simulink model "planta_controlador_integrados_rev_0"  (R2022a)
settings: Solver=ode1  StartTime=0.0  StopTime=tfinal  FixedStep=tstep  RelTol=1e-3
undefined symbols (not defined in the file or in its folder): wp_index_lim, wp_lat, wp_long, wp_time
settings Model: Creator=rodri  LastModifiedBy=rodri
settings DataIOCC: ExternalInput=[t2, u2]  SaveFormat=StructureWithTime  SignalLogging=off  DSMLogging=off  InspectSignalLogs=on  ReturnWorkspaceOutputs=off

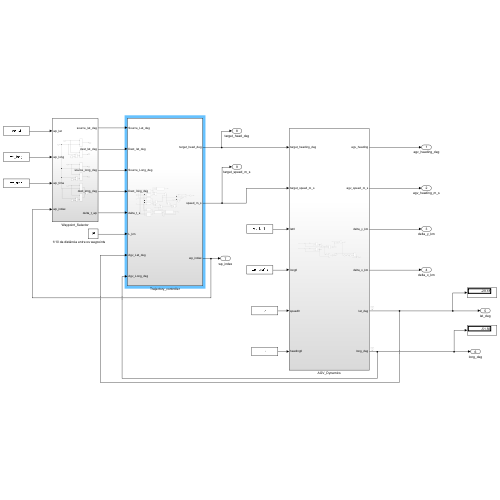
[thumbnail: Simulink's stored preview of the top-level diagram]
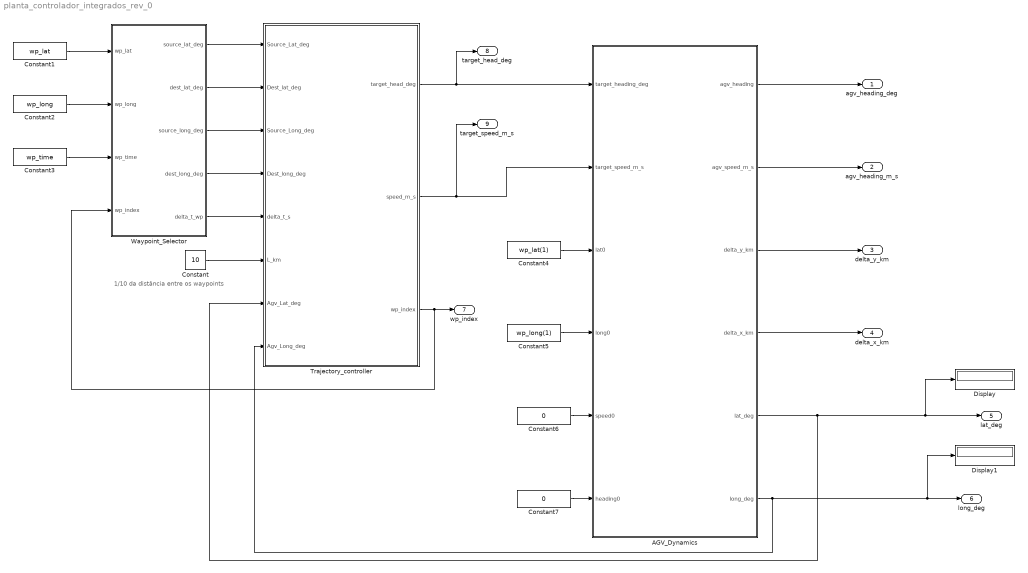
== system planta_controlador_integrados_rev_0 ==
  note: 1/10 da distância entre os waypoints
  AGV_Dynamics : Subsystem
  Constant : Constant  Value=10
  Constant1 : Constant  Value=wp_lat
  Constant2 : Constant  Value=wp_long
  Constant3 : Constant  Value=wp_time
  Constant4 : Constant  Value=wp_lat(1)
  Constant5 : Constant  Value=wp_long(1)
  Constant6 : Constant  Value=0
  Constant7 : Constant  Value=0
  Display : Display
  Display1 : Display
  Trajectory_controller : Subsystem
  Waypoint_Selector : Subsystem
  agv_heading_deg : Outport
  agv_heading_m_s : Outport  Port=2
  delta_y_km : Outport  Port=3
  delta_x_km : Outport  Port=4
  lat_deg : Outport  Port=5
  long_deg : Outport  Port=6
  wp_index : Outport  Port=7
  target_head_deg : Outport  Port=8
  target_speed_m_s : Outport  Port=9
  wires:
  Waypoint_Selector/1(source_lat_deg) -> Trajectory_controller/1(Source_Lat_deg)
  Waypoint_Selector/2(dest_lat_deg) -> Trajectory_controller/2(Dest_lat_deg)
  Waypoint_Selector/3(source_long_deg) -> Trajectory_controller/3(Source_Long_deg)
  Waypoint_Selector/4(dest_long_deg) -> Trajectory_controller/4(Dest_long_deg)
  Constant/1 -> Trajectory_controller/6(L_km)
  Constant1/1 -> Waypoint_Selector/1(wp_lat)
  Constant2/1 -> Waypoint_Selector/2(wp_long)
  Constant3/1 -> Waypoint_Selector/3(wp_time)
  Waypoint_Selector/5(delta_t_wp) -> Trajectory_controller/5(delta_t_s)
  Trajectory_controller/3(wp_index) -> Waypoint_Selector/4(wp_index), wp_index/1
  Trajectory_controller/1(target_head_deg) -> target_head_deg/1, AGV_Dynamics/1(target_heading_deg)
  Trajectory_controller/2(speed_m_s) -> AGV_Dynamics/2(target_speed_m_s), target_speed_m_s/1
  AGV_Dynamics/5(lat_deg) -> Display/1, lat_deg/1, Trajectory_controller/7(Agv_Lat_deg)
  AGV_Dynamics/6(long_deg) -> Display1/1, long_deg/1, Trajectory_controller/8(Agv_Long_deg)
  AGV_Dynamics/1(agv_heading) -> agv_heading_deg/1
  AGV_Dynamics/2(agv_speed_m_s) -> agv_heading_m_s/1
  AGV_Dynamics/3(delta_y_km) -> delta_y_km/1
  AGV_Dynamics/4(delta_x_km) -> delta_x_km/1
  Constant4/1 -> AGV_Dynamics/3(lat0)
  Constant5/1 -> AGV_Dynamics/4(long0)
  Constant6/1 -> AGV_Dynamics/5(speed0)
  Constant7/1 -> AGV_Dynamics/6(heading0)

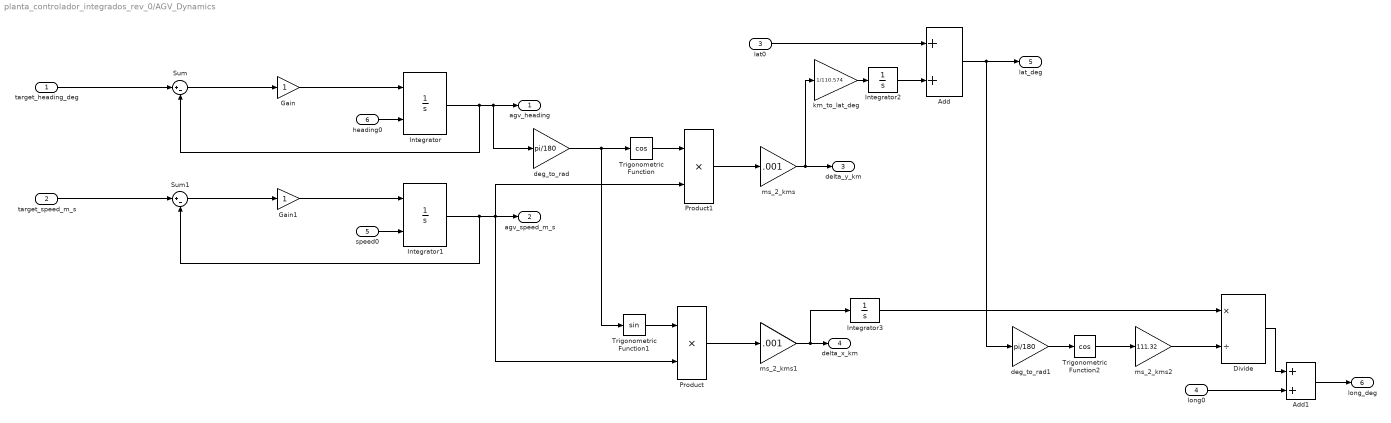
== system planta_controlador_integrados_rev_0/AGV_Dynamics ==
  target_heading_deg : Inport
  target_speed_m_s : Inport  Port=2
  lat0 : Inport  Port=3
  long0 : Inport  Port=4
  speed0 : Inport  Port=5
  heading0 : Inport  Port=6
  Add : Sum
  Add1 : Sum
  Divide : Product  Inputs=*/
  Gain : Gain
  Gain1 : Gain
  Integrator : Integrator  InitialConditionSource=external
  Integrator1 : Integrator  InitialConditionSource=external
  Integrator2 : Integrator
  Integrator3 : Integrator
  Product : Product
  Product1 : Product
  Sum : Sum  Inputs=|+-
  Sum1 : Sum  Inputs=|+-
  Trigonometric Function : Trigonometry  Operator=cos
  Trigonometric Function1 : Trigonometry
  Trigonometric Function2 : Trigonometry  Operator=cos
  deg_to_rad : Gain  Gain=pi/180
  deg_to_rad1 : Gain  Gain=pi/180
  km_to_lat_deg : Gain  Gain=1/110.574
  ms_2_kms : Gain  Gain=.001
  ms_2_kms1 : Gain  Gain=.001
  ms_2_kms2 : Gain  Gain=111.32
  agv_heading : Outport
  agv_speed_m_s : Outport  Port=2
  delta_y_km : Outport  Port=3
  delta_x_km : Outport  Port=4
  lat_deg : Outport  Port=5
  long_deg : Outport  Port=6
  wires:
  Integrator/1 -> Sum/2, deg_to_rad/1, agv_heading/1
  Gain/1 -> Integrator/1
  Sum/1 -> Gain/1
  target_heading_deg/1 -> Sum/1
  target_speed_m_s/1 -> Sum1/1
  Gain1/1 -> Integrator1/1
  Sum1/1 -> Gain1/1
  Integrator1/1 -> Sum1/2, Product1/2, Product/2, agv_speed_m_s/1
  heading0/1 -> Integrator/2
  speed0/1 -> Integrator1/2
  deg_to_rad/1 -> Trigonometric Function1/1, Trigonometric Function/1
  Trigonometric Function1/1 -> Product/1
  Product/1 -> ms_2_kms1/1
  Trigonometric Function/1 -> Product1/1
  Product1/1 -> ms_2_kms/1
  ms_2_kms/1 -> delta_y_km/1, km_to_lat_deg/1
  ms_2_kms1/1 -> Integrator3/1, delta_x_km/1
  lat0/1 -> Add/1
  km_to_lat_deg/1 -> Integrator2/1
  Add/1 -> deg_to_rad1/1, lat_deg/1
  deg_to_rad1/1 -> Trigonometric Function2/1
  Trigonometric Function2/1 -> ms_2_kms2/1
  long0/1 -> Add1/2
  Divide/1 -> Add1/1
  ms_2_kms2/1 -> Divide/2
  Add1/1 -> long_deg/1
  Integrator3/1 -> Divide/1
  Integrator2/1 -> Add/2

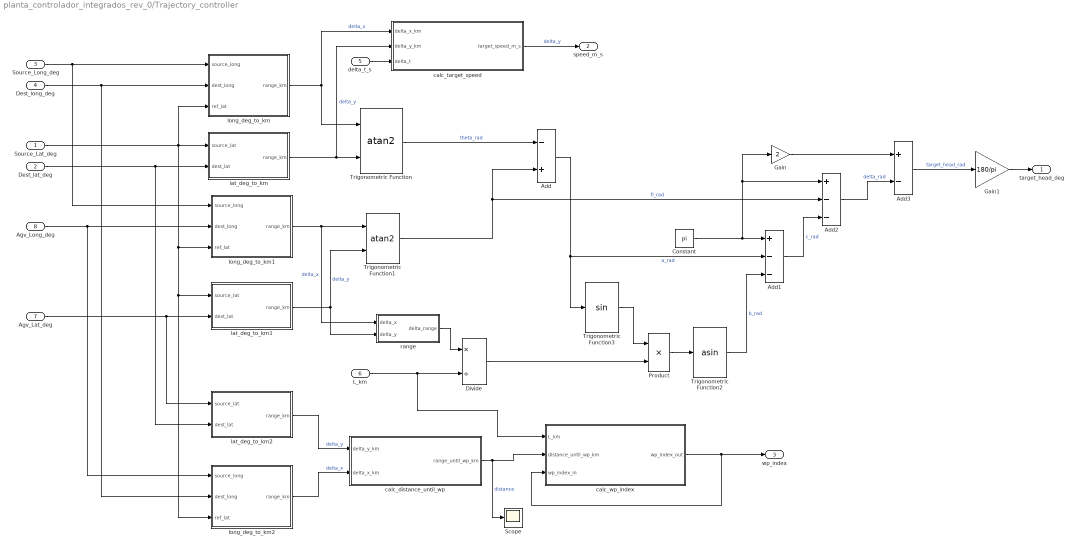
== system planta_controlador_integrados_rev_0/Trajectory_controller ==
  Source_Lat_deg : Inport
  Dest_lat_deg : Inport  Port=2
  Source_Long_deg : Inport  Port=3
  Dest_long_deg : Inport  Port=4
  delta_t_s : Inport  Port=5
  L_km : Inport  Port=6
  Agv_Lat_deg : Inport  Port=7
  Agv_Long_deg : Inport  Port=8
  Add : Sum  Inputs=-+
  Add1 : Sum  Inputs=+--
  Add2 : Sum  Inputs=+--
  Add3 : Sum  Inputs=+-
  Constant : Constant  Value=pi
  Divide : Product  Inputs=*/
  Gain : Gain  Gain=2
  Gain1 : Gain  Gain=180/pi
  Product : Product
  Scope : Scope
  Trigonometric Function : Trigonometry  Operator=atan2
  Trigonometric Function1 : Trigonometry  Operator=atan2
  Trigonometric Function2 : Trigonometry  Operator=asin
  Trigonometric Function3 : Trigonometry
  calc_distance_until_wp : Subsystem
  calc_target_speed : Subsystem
  calc_wp_index : Subsystem
  lat_deg_to_km : Subsystem
  lat_deg_to_km1 : Subsystem
  lat_deg_to_km2 : Subsystem
  long_deg_to_km : Subsystem
  long_deg_to_km1 : Subsystem
  long_deg_to_km2 : Subsystem
  range : Subsystem
  target_head_deg : Outport
  speed_m_s : Outport  Port=2
  wp_index : Outport  Port=3
  wires:
  Dest_lat_deg/1 -> lat_deg_to_km2/2(dest_lat), lat_deg_to_km/2(dest_lat)
  Source_Lat_deg/1 -> long_deg_to_km/3(ref_lat), long_deg_to_km2/3(ref_lat), lat_deg_to_km1/1(source_lat), long_deg_to_km1/3(ref_lat), lat_deg_to_km/1(source_lat)
  Agv_Lat_deg/1 -> lat_deg_to_km2/1(source_lat), lat_deg_to_km1/2(dest_lat)
  Source_Long_deg/1 -> long_deg_to_km1/1(source_long), long_deg_to_km/1(source_long)
  Dest_long_deg/1 -> long_deg_to_km/2(dest_long), long_deg_to_km2/2(dest_long)
  long_deg_to_km/1(range_km) -> calc_target_speed/1(delta_x_km), Trigonometric Function/1  "delta_x"
  lat_deg_to_km/1(range_km) -> calc_target_speed/2(delta_y_km), Trigonometric Function/2  "delta_y"
  Agv_Long_deg/1 -> long_deg_to_km2/1(source_long), long_deg_to_km1/2(dest_long)
  long_deg_to_km1/1(range_km) -> range/1(delta_x), Trigonometric Function1/1  "delta_x"
  lat_deg_to_km1/1(range_km) -> Trigonometric Function1/2, range/2(delta_y)  "delta_y"
  Trigonometric Function1/1 -> Add2/2, Add/2  "fi_rad"
  Trigonometric Function/1 -> Add/1  "theta_rad"
  Add/1 -> Add1/2, Trigonometric Function3/1  "a_rad"
  range/1(delta_range) -> Divide/1
  L_km/1 -> calc_wp_index/1(L_km), Divide/2
  Product/1 -> Trigonometric Function2/1
  Trigonometric Function3/1 -> Product/1
  Divide/1 -> Product/2
  Trigonometric Function2/1 -> Add1/3  "b_rad"
  Constant/1 -> Gain/1, Add2/1, Add1/1
  Add1/1 -> Add2/3  "c_rad"
  Add2/1 -> Add3/2  "delta_rad"
  Gain/1 -> Add3/1
  Add3/1 -> Gain1/1  "target_head_rad"
  Gain1/1 -> target_head_deg/1
  delta_t_s/1 -> calc_target_speed/3(delta_t)
  calc_target_speed/1(target_speed_m_s) -> speed_m_s/1  "delta_y"
  lat_deg_to_km2/1(range_km) -> calc_distance_until_wp/1(delta_y_km)  "delta_y"
  long_deg_to_km2/1(range_km) -> calc_distance_until_wp/2(delta_x_km)  "delta_x"
  calc_distance_until_wp/1(range_until_wp_km) -> Scope/1, calc_wp_index/2(distance_until_wp_km)  "distance"
  calc_wp_index/1(wp_index_out) -> calc_wp_index/3(wp_index_in), wp_index/1

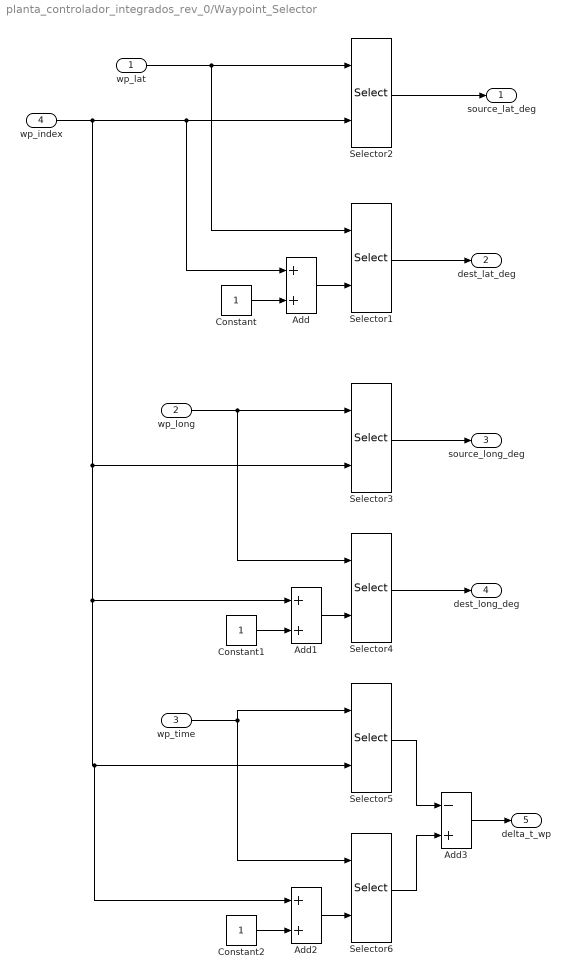
== system planta_controlador_integrados_rev_0/Waypoint_Selector ==
  wp_lat : Inport
  wp_long : Inport  Port=2
  wp_time : Inport  Port=3
  wp_index : Inport  Port=4
  Add : Sum
  Add1 : Sum
  Add2 : Sum
  Add3 : Sum  Inputs=-+
  Constant : Constant
  Constant1 : Constant
  Constant2 : Constant
  Selector{1..6} (6 alike) : Selector  InputPortWidth=num_of_wps  IndexOptions=Index vector (port)  Indices=[1 3]  OutputSizes=1
  source_lat_deg : Outport
  dest_lat_deg : Outport  Port=2
  source_long_deg : Outport  Port=3
  dest_long_deg : Outport  Port=4
  delta_t_wp : Outport  Port=5
  wires:
  Selector2/1 -> source_lat_deg/1
  Selector1/1 -> dest_lat_deg/1
  wp_lat/1 -> Selector2/1, Selector1/1
  Add/1 -> Selector1/2
  Constant/1 -> Add/2
  Selector3/1 -> source_long_deg/1
  Selector4/1 -> dest_long_deg/1
  wp_long/1 -> Selector4/1, Selector3/1
  Constant1/1 -> Add1/2
  Add1/1 -> Selector4/2
  Add2/1 -> Selector6/2
  Constant2/1 -> Add2/2
  wp_time/1 -> Selector5/1, Selector6/1
  wp_index/1 -> Add2/1, Selector5/2, Add1/1, Selector3/2, Selector2/2, Add/1
  Selector5/1 -> Add3/1
  Selector6/1 -> Add3/2
  Add3/1 -> delta_t_wp/1

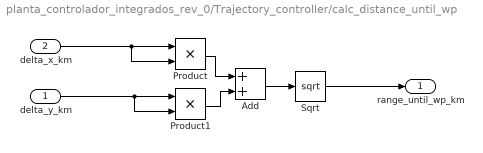
== system planta_controlador_integrados_rev_0/Trajectory_controller/calc_distance_until_wp ==
  delta_y_km : Inport
  delta_x_km : Inport  Port=2
  Add : Sum
  Product : Product
  Product1 : Product
  Sqrt : Sqrt
  range_until_wp_km : Outport
  wires:
  Sqrt/1 -> range_until_wp_km/1
  Product1/1 -> Add/2
  Product/1 -> Add/1
  Add/1 -> Sqrt/1
  delta_x_km/1 -> Product/1, Product/2
  delta_y_km/1 -> Product1/1, Product1/2

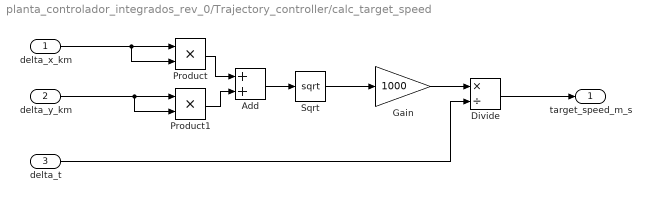
== system planta_controlador_integrados_rev_0/Trajectory_controller/calc_target_speed ==
  delta_x_km : Inport
  delta_y_km : Inport  Port=2
  delta_t : Inport  Port=3
  Add : Sum
  Divide : Product  Inputs=*/
  Gain : Gain  Gain=1000
  Product : Product
  Product1 : Product
  Sqrt : Sqrt
  target_speed_m_s : Outport
  wires:
  delta_y_km/1 -> Product1/2, Product1/1
  delta_x_km/1 -> Product/2, Product/1
  Add/1 -> Sqrt/1
  Product/1 -> Add/1
  Product1/1 -> Add/2
  Sqrt/1 -> Gain/1
  Gain/1 -> Divide/1
  delta_t/1 -> Divide/2
  Divide/1 -> target_speed_m_s/1

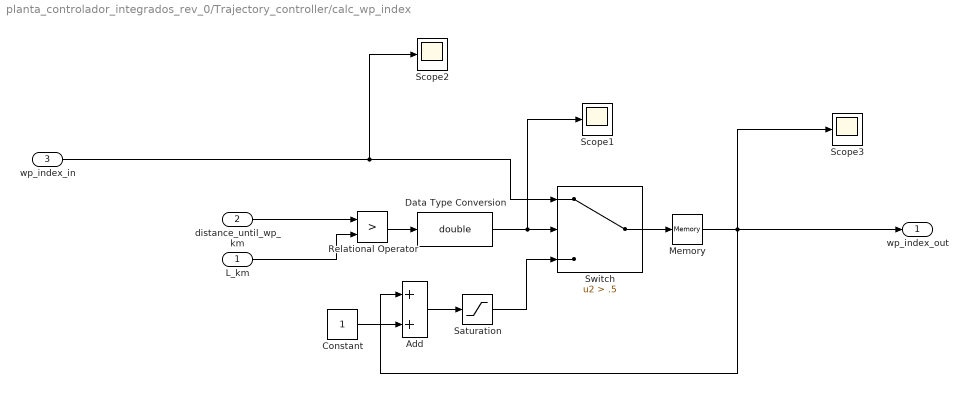
== system planta_controlador_integrados_rev_0/Trajectory_controller/calc_wp_index ==
  L_km : Inport
  distance_until_wp_km : Inport  Port=2
  wp_index_in : Inport  Port=3
  Add : Sum
  Constant : Constant
  Data Type Conversion : DataTypeConversion  OutDataTypeStr=double  SaturateOnIntegerOverflow=off  RndMeth=Floor
  Memory : Memory  InitialCondition=1
  Relational Operator : RelationalOperator  Operator=>  OutDataTypeStr=boolean  RndMeth=Simplest  InputSameDT=off
  Saturation : Saturate  UpperLimit=wp_index_lim  LowerLimit=1
  Scope1 : Scope
  Scope2 : Scope
  Scope3 : Scope
  Switch : Switch  Criteria=u2 > Threshold  Threshold=.5  SaturateOnIntegerOverflow=off  InputSameDT=off
  wp_index_out : Outport
  wires:
  distance_until_wp_km/1 -> Relational Operator/1
  L_km/1 -> Relational Operator/2
  Relational Operator/1 -> Data Type Conversion/1
  Data Type Conversion/1 -> Scope1/1, Switch/2
  Switch/1 -> Memory/1
  Memory/1 -> Add/1, Scope3/1, wp_index_out/1
  wp_index_in/1 -> Scope2/1, Switch/1
  Add/1 -> Saturation/1
  Constant/1 -> Add/2
  Saturation/1 -> Switch/3

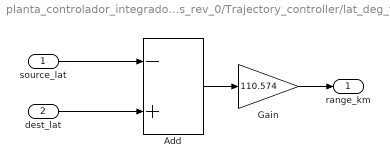
== system planta_controlador_integrados_rev_0/Trajectory_controller/lat_deg_to_km ==
  source_lat : Inport
  dest_lat : Inport  Port=2
  Add : Sum  Inputs=-+
  Gain : Gain  Gain=110.574
  range_km : Outport
  wires:
  source_lat/1 -> Add/1
  dest_lat/1 -> Add/2
  Add/1 -> Gain/1
  Gain/1 -> range_km/1

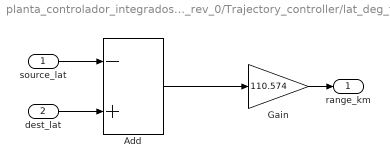
== system planta_controlador_integrados_rev_0/Trajectory_controller/lat_deg_to_km1 ==
  source_lat : Inport
  dest_lat : Inport  Port=2
  Add : Sum  Inputs=-+
  Gain : Gain  Gain=110.574
  range_km : Outport
  wires:
  source_lat/1 -> Add/1
  dest_lat/1 -> Add/2
  Add/1 -> Gain/1
  Gain/1 -> range_km/1

== system planta_controlador_integrados_rev_0/Trajectory_controller/lat_deg_to_km2 ==
  source_lat : Inport
  dest_lat : Inport  Port=2
  Add : Sum  Inputs=-+
  Gain : Gain  Gain=110.574
  range_km : Outport
  wires:
  Gain/1 -> range_km/1
  Add/1 -> Gain/1
  dest_lat/1 -> Add/2
  source_lat/1 -> Add/1

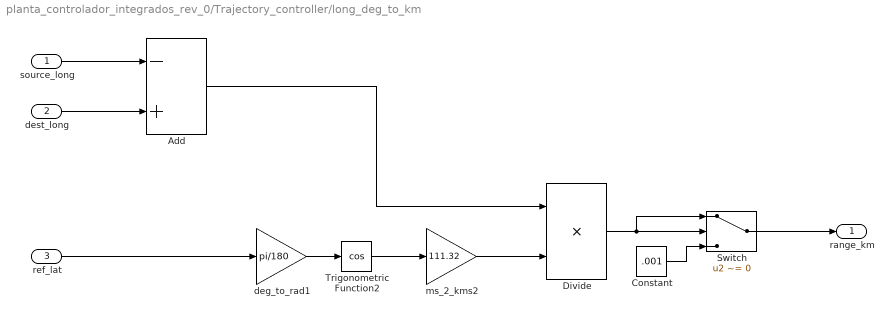
== system planta_controlador_integrados_rev_0/Trajectory_controller/long_deg_to_km ==
  source_long : Inport
  dest_long : Inport  Port=2
  ref_lat : Inport  Port=3
  Add : Sum  Inputs=-+
  Constant : Constant  Value=.001
  Divide : Product  Inputs=**
  Switch : Switch  Criteria=u2 ~= 0  SaturateOnIntegerOverflow=off  InputSameDT=off
  Trigonometric Function2 : Trigonometry  Operator=cos
  deg_to_rad1 : Gain  Gain=pi/180
  ms_2_kms2 : Gain  Gain=111.32
  range_km : Outport
  wires:
  Add/1 -> Divide/1
  dest_long/1 -> Add/2
  source_long/1 -> Add/1
  Trigonometric Function2/1 -> ms_2_kms2/1
  deg_to_rad1/1 -> Trigonometric Function2/1
  ms_2_kms2/1 -> Divide/2
  Divide/1 -> Switch/1, Switch/2
  ref_lat/1 -> deg_to_rad1/1
  Switch/1 -> range_km/1
  Constant/1 -> Switch/3

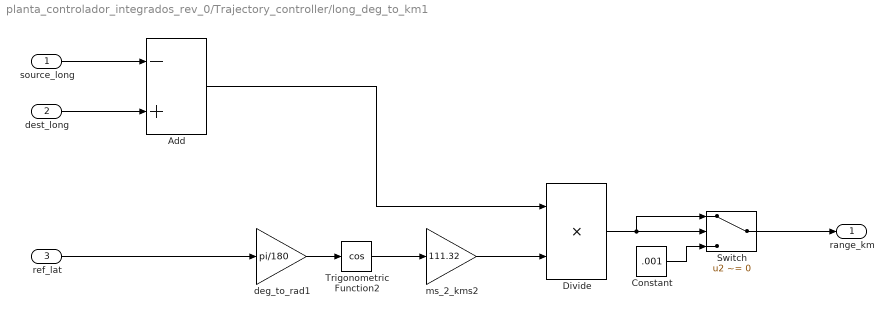
== system planta_controlador_integrados_rev_0/Trajectory_controller/long_deg_to_km1 ==
  source_long : Inport
  dest_long : Inport  Port=2
  ref_lat : Inport  Port=3
  Add : Sum  Inputs=-+
  Constant : Constant  Value=.001
  Divide : Product  Inputs=**
  Switch : Switch  Criteria=u2 ~= 0  SaturateOnIntegerOverflow=off  InputSameDT=off
  Trigonometric Function2 : Trigonometry  Operator=cos
  deg_to_rad1 : Gain  Gain=pi/180
  ms_2_kms2 : Gain  Gain=111.32
  range_km : Outport
  wires:
  Constant/1 -> Switch/3
  Switch/1 -> range_km/1
  ref_lat/1 -> deg_to_rad1/1
  Divide/1 -> Switch/2, Switch/1
  ms_2_kms2/1 -> Divide/2
  deg_to_rad1/1 -> Trigonometric Function2/1
  Trigonometric Function2/1 -> ms_2_kms2/1
  source_long/1 -> Add/1
  dest_long/1 -> Add/2
  Add/1 -> Divide/1

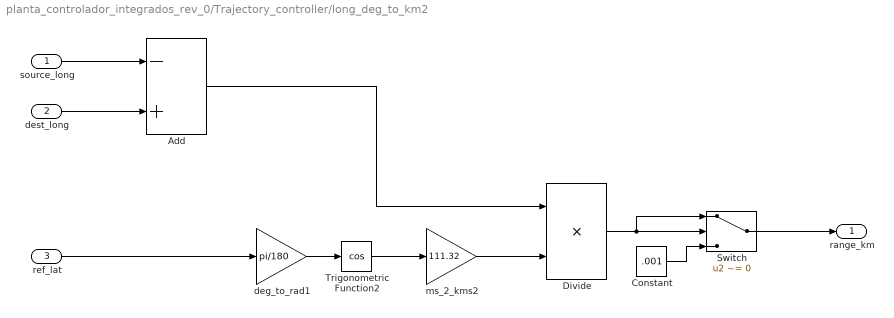
== system planta_controlador_integrados_rev_0/Trajectory_controller/long_deg_to_km2 ==
  source_long : Inport
  dest_long : Inport  Port=2
  ref_lat : Inport  Port=3
  Add : Sum  Inputs=-+
  Constant : Constant  Value=.001
  Divide : Product  Inputs=**
  Switch : Switch  Criteria=u2 ~= 0  SaturateOnIntegerOverflow=off  InputSameDT=off
  Trigonometric Function2 : Trigonometry  Operator=cos
  deg_to_rad1 : Gain  Gain=pi/180
  ms_2_kms2 : Gain  Gain=111.32
  range_km : Outport
  wires:
  Constant/1 -> Switch/3
  Switch/1 -> range_km/1
  ref_lat/1 -> deg_to_rad1/1
  Divide/1 -> Switch/2, Switch/1
  ms_2_kms2/1 -> Divide/2
  deg_to_rad1/1 -> Trigonometric Function2/1
  Trigonometric Function2/1 -> ms_2_kms2/1
  source_long/1 -> Add/1
  dest_long/1 -> Add/2
  Add/1 -> Divide/1

== system planta_controlador_integrados_rev_0/Trajectory_controller/range ==
  delta_x : Inport
  delta_y : Inport  Port=2
  MATLAB Function : MATLAB Function  TreatAsAtomicUnit=on
  delta_range : Outport
  wires:
  MATLAB Function/1(delta_range) -> delta_range/1  "delta_range"
  delta_x/1 -> MATLAB Function/1(delta_x)  "delta_x"
  delta_y/1 -> MATLAB Function/2(delta_y)  "delta_y"

== matlab function planta_controlador_integrados_rev_0/Trajectory_controller/range/MATLAB Function ==
  data: delta_x input; delta_range output; delta_y input
function delta_range = range(delta_x, delta_y)

delta_range = sqrt(delta_x^2 + delta_y*2);
